simulink model "QuadcopterSimModel_INDI_Traj"  (R2018b)
settings: Solver=ode23  StartTime=0.0  StopTime=1000  FixedStep=sample_time  RelTol=1e-4  EnableMultiTasking=on
undefined symbols (not defined in the file): alt_ground, atmosphere, cycle, DiscIntNeverNeededParam, envir, fm_loiter, g, jystck, pos_ref, sigbuilder_block, traj_empty, waypoints, wind
libraries: simulink x6, ndi_lib x5, filters_lib x5, axes_transformation_lib x4, angles_lib x3, unit_conversions_lib x3, cntrl_atti_red_indi_lib x2, traj_lib x2, aerolibfltsims x2, control_allocation_lib x1, sensors_lib x1, atmosphere_lib x1
(part 1 of 3)
settings Model: Creator=Yannic  LastModifiedBy=eike
settings SolverCC: ZeroCrossControl=DisableAll
settings DataIOCC: LimitDataPoints=on  ReturnWorkspaceOutputs=on
settings OptimizationCC: EfficientMapNaN2IntZero=off  LifeSpan=inf
settings DebuggingCC: ReadBeforeWriteMsg=DisableAll  WriteAfterWriteMsg=DisableAll  WriteAfterReadMsg=DisableAll  MultiTaskDSMMsg=none  AllowSymbolicDim=off  LibraryContextMissingDiagnostic=none  SFUnexpectedBacktrackingDiag=warning  SFNoUnconditionalDefaultTransitionDiag=warning  SFExecutionAtInitializationDiag=none
settings HardwareCC: TargetBitPerLong=64  TargetBitPerPointer=64  TargetBitPerSizeT=64  TargetBitPerPtrDiffT=64  TargetLongLongMode=on  TargetIntDivRoundTo=Zero  TargetEndianess=LittleEndian  TargetWordSize=64  TargetHWDeviceType=MATLAB Host  ProdEqTarget=off
settings ModelReferenceCC: UpdateModelReferenceTargets=IfOutOfDate  PropagateSignalLabelsOutOfModel=off
settings SFSimCC: SFSimEcho=off  SimUseLocalCustomCode=off
settings CodeAppCC: MaxIdLength=128
settings GRTTargetCC: TargetLangStandard=C89/C90 (ANSI)  CombineOutputUpdateFcns=off  GRTInterface=on
settings ConfigComp: CovMetricSettings=dw  CovHtmlReporting=on  CovSaveCumulativeToWorkspaceVar=on  CovSaveSingleToWorkspaceVar=on  CovExternalEMLEnable=off

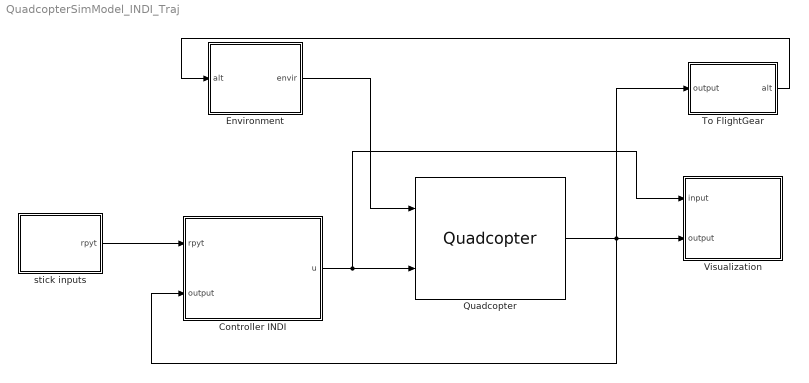
== system QuadcopterSimModel_INDI_Traj ==
  Controller INDI : Subsystem
  Environment : Subsystem
  Quadcopter : quadcopter_lib/Quadcopter  copter_=copter  IC_=IC  grnd_=grnd
      settings: SourceProductName=LADAC
  To FlightGear : Subsystem
  Visualization : Subsystem
  stick inputs : Subsystem
  wires:
  Environment/1(envir) -> Quadcopter/1
  Quadcopter/1 -> To FlightGear/1(output), Visualization/2(output), Controller INDI/2(output)
  To FlightGear/1(alt) -> Environment/1(alt)
  Controller INDI/1(u) -> Quadcopter/2, Visualization/1(input)
  stick inputs/1(rpyt) -> Controller INDI/1(rpyt)

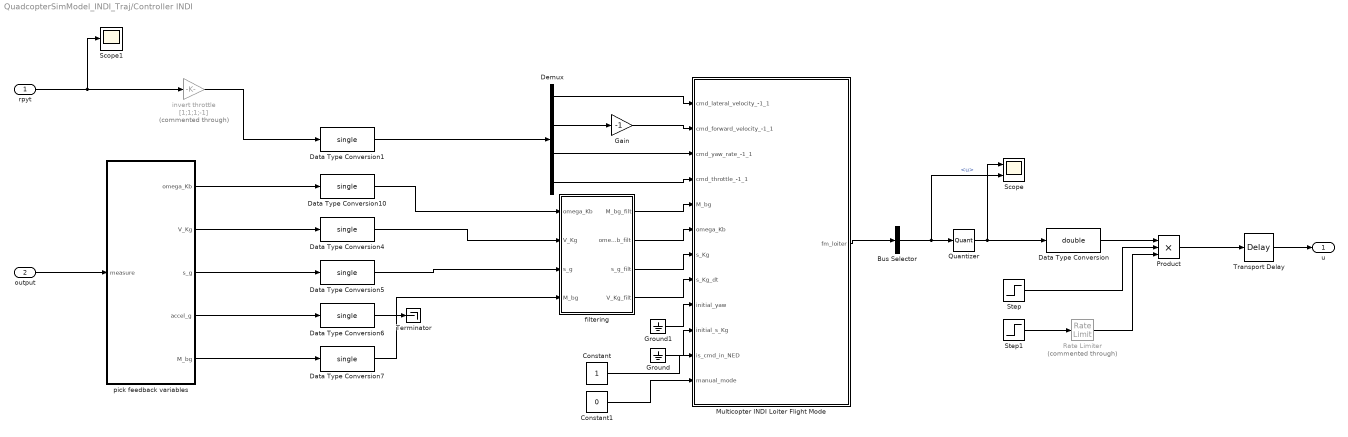
== system QuadcopterSimModel_INDI_Traj/Controller INDI ==
  rpyt : Inport  OutDataTypeStr=double
  output : Inport  Port=2
  Bus Selector : BusSelector  OutputSignals=fm_alt_hold.u
  Constant : Constant
  Constant1 : Constant  Value=0  OutDataTypeStr=single
  Data Type Conversion : DataTypeConversion  OutDataTypeStr=double
  Data Type Conversion{1,4..7,10} (6 alike) : DataTypeConversion  OutDataTypeStr=single
  Demux : Demux
  Gain : Gain  Gain=-1
  Ground : Ground
  Ground1 : Ground
  Multicopter INDI Loiter Flight Mode : Subsystem  AncestorBlock=fm_copter_loiter_indi_lib/Multicopter INDI Loiter Flight Mode  mask{fm=fm_loiter}
      mask prompts: fm "Multicopter INDI loiter flight  struct"
      mask DialogControl DescGroupVar Prompt: Multicopter INDI Loiter Flight Mode
      mask DialogControl DescTextVar Prompt: Loiter flight mode using the reduced attitude controller with INDI.
      mask DialogControl Control2 Prompt: To intialize the parameters struct see multicopterFlightModeLoiter.
  Product : Product  Inputs=3
  Quantizer : Quantizer  QuantizationInterval=0.001
  Rate Limiter : RateLimiter  Commented=through  SampleTimeMode=inherited  InitialCondition=1
  Scope : Scope  NumInputPorts=2
  Scope1 : Scope
  Step : Step  Time=100  Before=[1;1;1;1]  After=[1;1;1;1]  SampleTime=0
  Step1 : Step  Time=5  Before=[1;1;1;1]  After=[1;1;1;1]  SampleTime=0
  Terminator : Terminator
  Transport Delay : TransportDelay  DelayTime=0.01*0
  filtering : Subsystem
  invert throttle : Gain  Commented=through  Gain=[1;1;1;-1]
  pick feedback variables : Subsystem
  u : Outport  OutDataTypeStr=double  PortDimensions=4
  wires:
  pick feedback variables/1(omega_Kb) -> Data Type Conversion10/1
  output/1 -> pick feedback variables/1(measure)
  rpyt/1 -> invert throttle/1, Scope1/1
  Bus Selector/1 -> Scope/2, Quantizer/1  "<u>"
  pick feedback variables/3(s_g) -> Data Type Conversion5/1
  Data Type Conversion6/1 -> Terminator/1
  pick feedback variables/4(accel_g) -> Data Type Conversion6/1
  pick feedback variables/2(V_Kg) -> Data Type Conversion4/1
  Transport Delay/1 -> u/1
  Step/1 -> Product/2
  Data Type Conversion/1 -> Product/1
  Product/1 -> Transport Delay/1
  Rate Limiter/1 -> Product/3
  Data Type Conversion1/1 -> Demux/1
  pick feedback variables/5(M_bg) -> Data Type Conversion7/1
  Ground/1 -> Multicopter INDI Loiter Flight Mode/10(initial_s_Kg)
  Step1/1 -> Rate Limiter/1
  invert throttle/1 -> Data Type Conversion1/1
  Multicopter INDI Loiter Flight Mode/1(fm_loiter) -> Bus Selector/1
  Demux/4 -> Multicopter INDI Loiter Flight Mode/4(cmd_throttle_-1_1)
  Demux/3 -> Multicopter INDI Loiter Flight Mode/3(cmd_yaw_rate_-1_1)
  Constant/1 -> Multicopter INDI Loiter Flight Mode/11(is_cmd_in_NED)
  Ground1/1 -> Multicopter INDI Loiter Flight Mode/9(initial_yaw)
  Demux/2 -> Gain/1
  Demux/1 -> Multicopter INDI Loiter Flight Mode/1(cmd_lateral_velocity_-1_1)
  Gain/1 -> Multicopter INDI Loiter Flight Mode/2(cmd_forward_velocity_-1_1)
  Data Type Conversion10/1 -> filtering/1(omega_Kb)
  Data Type Conversion4/1 -> filtering/2(V_Kg)
  Data Type Conversion5/1 -> filtering/3(s_g)
  Data Type Conversion7/1 -> filtering/4(M_bg)
  filtering/1(M_bg_filt) -> Multicopter INDI Loiter Flight Mode/5(M_bg)
  filtering/2(omega_Kb_filt) -> Multicopter INDI Loiter Flight Mode/6(omega_Kb)
  filtering/3(s_g_filt) -> Multicopter INDI Loiter Flight Mode/7(s_Kg)
  filtering/4(V_Kg_filt) -> Multicopter INDI Loiter Flight Mode/8(s_Kg_dt)
  Quantizer/1 -> Scope/1, Data Type Conversion/1
  Constant1/1 -> Multicopter INDI Loiter Flight Mode/12(manual_mode)

== system QuadcopterSimModel_INDI_Traj/Environment ==
  alt : Inport
  Bus Assignment : BusAssignment  AssignedSignals=atmosphere,wind,g,alt_ground
  Bus Creator : BusCreator  Inputs=2
  Constant1 : Constant  Value=envir  OutDataTypeStr=Bus: envirBus
  Constant2 : Constant  Value=zeros(3,1)
  Constant3 : Constant  Value=envir.g
  From FlightGear : Subsystem
  Gain : Gain  Gain=0
  ISA Atmosphere Model : atmosphere_lib/ISA Atmosphere Model  SystemSampleTime=-1
      settings: SourceProductName=LADAC
  Rate Transition{,1..4} (5 alike) : RateTransition
  Step : Step  Time=5  After=[0;10;0]  SampleTime=0
  envir : Outport
  wires:
  From FlightGear/1(h_ground) -> Rate Transition1/1  "h"
  Rate Transition2/1 -> Bus Assignment/3
  Rate Transition3/1 -> Bus Assignment/2
  Bus Assignment/1 -> envir/1
  Rate Transition/1 -> Bus Assignment/1
  ISA Atmosphere Model/1 -> Rate Transition3/1
  Step/1 -> Gain/1  "V_Wg"
  Rate Transition1/1 -> Bus Assignment/5
  Constant1/1 -> Rate Transition/1
  alt/1 -> ISA Atmosphere Model/1
  Bus Creator/1 -> Rate Transition2/1
  Constant2/1 -> Bus Creator/2  "V_Wg_dt"
  Rate Transition4/1 -> Bus Assignment/4
  Constant3/1 -> Rate Transition4/1
  Gain/1 -> Bus Creator/1

== system QuadcopterSimModel_INDI_Traj/To FlightGear ==
  output : Inport
  Bus Selector1 : BusSelector  OutputSignals=rigidBodyBus.s_g_in_m,rigidBodyBus.EulerAngles_in_rad,motorBus.angular_velocity_in_rad_per_s
  Compare To Constant : simulink/Logic and Bit Operations/Compare To Constant  relop=<=  const=2*pi*1000  OutDataTypeStr=boolean
  Constant : Constant  Value=4
  Flight Gear Animation (Quadcopter) : flightgear_visualization_lib/Flight Gear Animation (Quadcopter)  inital_lat=pos_ref.lat  inital_long=pos_ref.lon  inital_height=pos_ref.alt  remoteURL=fg.remoteURL  remotePort=fg.remotePort
      settings: SourceProductName=LADAC
  Ground : Ground
  Integrator : Integrator  ExternalReset=rising
  Selector : Selector  InputPortWidth=3  IndexOptions=Index vector (dialog)  Indices=3  OutputSizes=1
  Unit Delay : UnitDelay  SampleTime=-1
  geographic position : Subsystem
  rad2deg : unit_conversions_lib/rad2deg
      settings: SourceProductName=LADAC
  alt : Outport
  wires:
  Bus Selector1/1 -> geographic position/1(s_E), Flight Gear Animation (Quadcopter)/1  "<s_g_in_m>"
  output/1 -> Bus Selector1/1
  geographic position/1(lat,lon,alt) -> Selector/1
  Bus Selector1/2 -> Flight Gear Animation (Quadcopter)/2  "<EulerAngles_in_rad>"
  Bus Selector1/3 -> rad2deg/1  "<angular_velocity_in_rad_per_s>"
  Selector/1 -> alt/1
  Constant/1 -> Flight Gear Animation (Quadcopter)/3
  Ground/1 -> Flight Gear Animation (Quadcopter)/4
  Integrator/1 -> Unit Delay/1, Flight Gear Animation (Quadcopter)/5
  Unit Delay/1 -> Compare To Constant/1
  Compare To Constant/1 -> Integrator/2
  rad2deg/1 -> Integrator/1

== system QuadcopterSimModel_INDI_Traj/Visualization ==
  input : Inport
  output : Inport  Port=2
  Aerodynamics : Subsystem
  Bus Selector : BusSelector  OutputSignals=rigidBodyBus,aeroBus,propulsionBus,motorBus
  Motor : Subsystem
  Propulsion : Subsystem
  Scope : Scope
  rigid_body : Subsystem
  wires:
  output/1 -> Bus Selector/1
  Bus Selector/1 -> rigid_body/1(rigidBodyBus)  "<rigidBodyBus>"
  Bus Selector/2 -> Aerodynamics/1(aeroBus)  "<aeroBus>"
  Bus Selector/3 -> Propulsion/1(propulsionBus)  "<propulsionBus>"
  Bus Selector/4 -> Motor/1(motorBus)  "<motorBus>"
  input/1 -> Scope/1

== system QuadcopterSimModel_INDI_Traj/stick inputs ==
  Calibrated Joystick : joystick_lib/Calibrated Joystick  jystck=jystck
      settings: SourceProductName=LADAC
  Constant1 : Constant  Value=jystck.enable
  Scope : Scope
  Selector2 : Selector  InputPortWidth=8  IndexOptions=Index vector (dialog)  Indices=[1,2,3,4]  OutputSizes=1
  Signal builder : Subsystem
  Switch1 : Switch  Criteria=u2 > Threshold
  rpyt : Outport
  wires:
  Signal builder/1(r) -> Switch1/3
  Switch1/1 -> Selector2/1, Scope/1
  Constant1/1 -> Calibrated Joystick/Enable, Switch1/2
  Calibrated Joystick/1 -> Switch1/1
  Selector2/1 -> rpyt/1

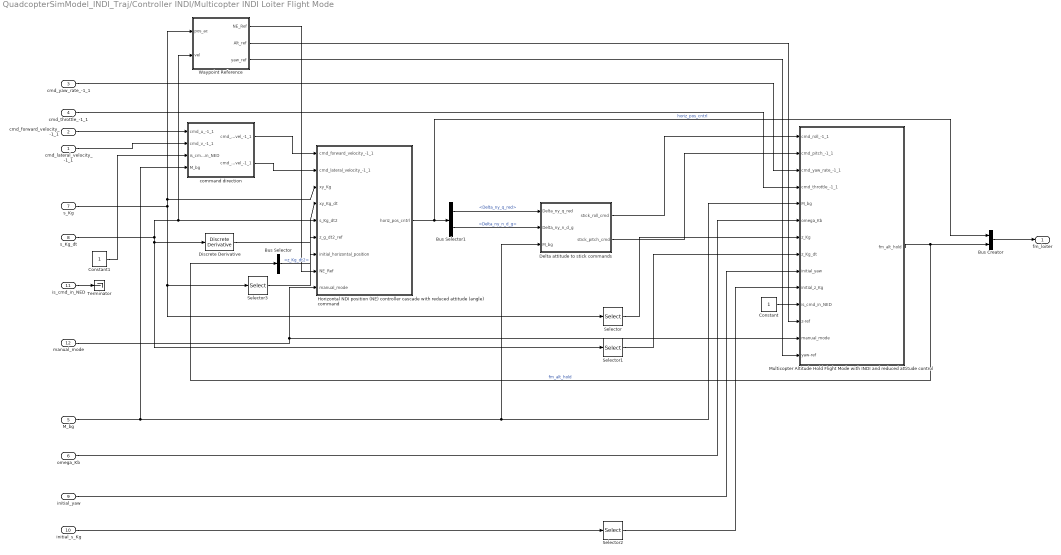
== system QuadcopterSimModel_INDI_Traj/Controller INDI/Multicopter INDI Loiter Flight Mode ==
  cmd_lateral_velocity_-1_1 : Inport  SampleTime=fm.sample_time
  cmd_forward_velocity_-1_1 : Inport  Port=2  SampleTime=fm.sample_time
  cmd_yaw_rate_-1_1 : Inport  Port=3  SampleTime=fm.sample_time
  cmd_throttle_-1_1 : Inport  Port=4  SampleTime=fm.sample_time
  M_bg : Inport  Port=5  SampleTime=fm.sample_time
  omega_Kb : Inport  Port=6  SampleTime=fm.sample_time
  s_Kg : Inport  Port=7  SampleTime=fm.sample_time
  s_Kg_dt : Inport  Port=8  SampleTime=fm.sample_time
  initial_yaw : Inport  Port=9  SampleTime=fm.sample_time
  initial_s_Kg : Inport  Port=10  SampleTime=fm.sample_time
  is_cmd_in_NED : Inport  Port=11  SampleTime=fm.sample_time
  manual_mode : Inport  Port=12
  Bus Creator : BusCreator  Inputs=2
  Bus Selector : BusSelector  OutputSignals=alt_cntrl.reference.z_Kg_dt2
  Bus Selector1 : BusSelector  OutputSignals=pseudo_control.Delta_ny_q_red,pseudo_control.Delta_ny_n_d_g
  Constant : Constant
  Constant1 : Constant  OutDataTypeStr=Inherit: Inherit via back propagation
  Delta attitude to stick commands : Subsystem
  Discrete Derivative : simulink/Discrete/Discrete Derivative  gainval=1.0  ICPrevScaledInput=0.0  OutMin=[]  OutMax=[]  OutDataType=fixdt(1, 16)  OutScaling=2^-10  DoSatur=off
  Horizontal NDI position (NE) controller cascade with reduced attitude (angle) command : Subsystem  AncestorBlock=|  mask{horiz_pos_cntrl=fm.horiz_pos_cntrl, T=2./fm.fm_alt.cntrl.atti_cntrl.rm.lean.omega + fm.fm_alt.motor_time_constant + 2./fm.fm_alt.sens_filt.omega}
      | cntrl_horiz_pos_indi_lib/Horizontal NDI position (NE) controller cascade
      | with reduced attitude (angle) command
      mask prompts: horiz_pos_cntrl "horizontal position controller struct"; T "inner loop time constant"
      mask DialogControl DescGroupVar Prompt: Horizontal position controller cascade
      mask DialogControl DescTextVar Prompt: The commanded velocity is filtered and the control error is converted into desired accerlations in x_g and y_g direction. The commanded accelerations are converted into commanded to reduced attitude angles.
      mask DialogControl Control2 Prompt: To initialize a horizontal position controller parameters struct see cntrlHorizPosIndiLoadParams
  Multicopter Altitude Hold Flight Mode with INDI and reduced attitude control : Subsystem  AncestorBlock=fm_copter_alt_hold_indi_lib/Multicopter Altitude Hold Flight Mode with INDI and reduced attitude control  mask{fm=fm.fm_alt}
      mask prompts: fm "Multicopter Altitude Hold Flight Mode (INDI) struct"
      mask DialogControl DescGroupVar Prompt: Multicopter Attitude Flight Mode with INDI and reduced attitude control
      mask DialogControl DescTextVar Prompt: Controller is basically implemented according to [1]
      mask DialogControl Control2 Prompt: [1] Sun, S., Baert, M., Van Schijndel, B. S., & De Visser, C. (2020, May). Upset Recovery Control for Quadrotors Subjected to a Complete Rotor Failure from Large Initial Disturbances. In 2020 IEEE International Conference on Robotics and Automation (ICRA) (pp. 4273-4279). IEEE.
      mask DialogControl Control3 Prompt: To initialize an altitude hold flight mode struct see fmCopterAltHoldIndiLoadParams
  Selector : Selector  InputPortWidth=3  IndexOptions=Index vector (dialog)  Indices=3  OutputSizes=1
  Selector1 : Selector  InputPortWidth=3  IndexOptions=Index vector (dialog)  Indices=3  OutputSizes=1
  Selector2 : Selector  InputPortWidth=3  IndexOptions=Index vector (dialog)  Indices=3  OutputSizes=1
  Selector3 : Selector  InputPortWidth=3  IndexOptions=Index vector (dialog)  Indices=[1,2]  OutputSizes=1
  Terminator : Terminator
  Waypoint Reference : Subsystem
  command direction : Subsystem
  fm_loiter : Outport  OutDataTypeStr=single  SampleTime=fm.sample_time
  wires:
  is_cmd_in_NED/1 -> Terminator/1
  command direction/2(cmd_east_vel_-1_1) -> Horizontal NDI position (NE) controller cascade with reduced attitude (angle) command/2(cmd_lateral_velocity_-1_1)
  command direction/1(cmd_north_vel_-1_1) -> Horizontal NDI position (NE) controller cascade with reduced attitude (angle) command/1(cmd_forward_velocity_-1_1)
  Bus Creator/1 -> fm_loiter/1
  Bus Selector1/1 -> Delta attitude to stick commands/1(Delta_ny_q_red)  "<Delta_ny_q_red>"
  Selector2/1 -> Multicopter Altitude Hold Flight Mode with INDI and reduced attitude control/10(initial_z_Kg)
  Constant1/1 -> command direction/3(is_cmd_in_NED)
  Delta attitude to stick commands/1(stick_roll_cmd) -> Multicopter Altitude Hold Flight Mode with INDI and reduced attitude control/1(cmd_roll_-1_1)
  Selector/1 -> Multicopter Altitude Hold Flight Mode with INDI and reduced attitude control/7(z_Kg)
  cmd_lateral_velocity_-1_1/1 -> command direction/2(cmd_v_-1_1)
  Bus Selector/1 -> Horizontal NDI position (NE) controller cascade with reduced attitude (angle) command/6(z_g_dt2_ref)  "<z_Kg_dt2>"
  cmd_throttle_-1_1/1 -> Multicopter Altitude Hold Flight Mode with INDI and reduced attitude control/4(cmd_throttle_-1_1)
  initial_yaw/1 -> Multicopter Altitude Hold Flight Mode with INDI and reduced attitude control/9(initial_yaw)
  Delta attitude to stick commands/2(stick_pitch_cmd) -> Multicopter Altitude Hold Flight Mode with INDI and reduced attitude control/2(cmd_pitch_-1_1)
  s_Kg/1 -> Selector/1, Selector3/1, Waypoint Reference/1(pos_ac), Horizontal NDI position (NE) controller cascade with reduced attitude (angle) command/3(xy_Kg)
  Selector1/1 -> Multicopter Altitude Hold Flight Mode with INDI and reduced attitude control/8(z_Kg_dt)
  Multicopter Altitude Hold Flight Mode with INDI and reduced attitude control/1(fm_alt_hold) -> Bus Selector/1, Bus Creator/2  "fm_alt_hold"
  M_bg/1 -> command direction/4(M_bg), Multicopter Altitude Hold Flight Mode with INDI and reduced attitude control/5(M_bg), Delta attitude to stick commands/3(M_bg)
  Bus Selector1/2 -> Delta attitude to stick commands/2(Delta_ny_n_d_g)  "<Delta_ny_n_d_g>"
  Horizontal NDI position (NE) controller cascade with reduced attitude (angle) command/1(horiz_pos_cntrl) -> Bus Selector1/1, Bus Creator/1  "horiz_pos_cntrl"
  omega_Kb/1 -> Multicopter Altitude Hold Flight Mode with INDI and reduced attitude control/6(omega_Kb)
  initial_s_Kg/1 -> Selector2/1
  Selector3/1 -> Horizontal NDI position (NE) controller cascade with reduced attitude (angle) command/7(initial_horizontal_position)
  Constant/1 -> Multicopter Altitude Hold Flight Mode with INDI and reduced attitude control/11(is_cmd_in_NED)
  cmd_yaw_rate_-1_1/1 -> Multicopter Altitude Hold Flight Mode with INDI and reduced attitude control/3(cmd_yaw_rate_-1_1)
  Discrete Derivative/1 -> Horizontal NDI position (NE) controller cascade with reduced attitude (angle) command/5(s_Kg_dt2)
  s_Kg_dt/1 -> Selector1/1, Discrete Derivative/1, Horizontal NDI position (NE) controller cascade with reduced attitude (angle) command/4(xy_Kg_dt), Waypoint Reference/2(vel)
  cmd_forward_velocity_-1_1/1 -> command direction/1(cmd_u_-1_1)
  Waypoint Reference/1(NE_Ref) -> Horizontal NDI position (NE) controller cascade with reduced attitude (angle) command/8(NE_Ref)
  manual_mode/1 -> Horizontal NDI position (NE) controller cascade with reduced attitude (angle) command/9(manual_mode), Multicopter Altitude Hold Flight Mode with INDI and reduced attitude control/13(manual_mode)
  Waypoint Reference/2(Alt_ref) -> Multicopter Altitude Hold Flight Mode with INDI and reduced attitude control/12(z-ref)
  Waypoint Reference/3(yaw_ref) -> Multicopter Altitude Hold Flight Mode with INDI and reduced attitude control/14(yaw-ref)

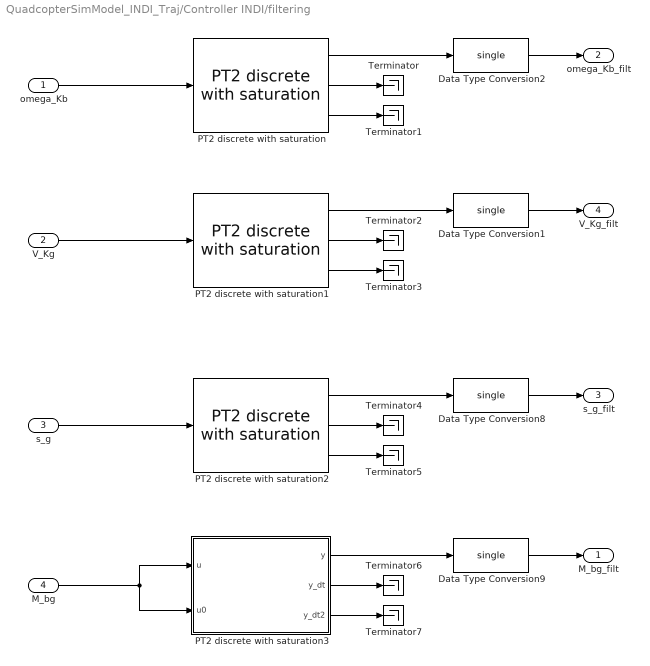
== system QuadcopterSimModel_INDI_Traj/Controller INDI/filtering ==
  omega_Kb : Inport
  V_Kg : Inport  Port=2
  s_g : Inport  Port=3
  M_bg : Inport  Port=4
  Data Type Conversion{1..2,8..9} (4 alike) : DataTypeConversion  OutDataTypeStr=single
  PT2 discrete with saturation : filters_lib/PT2 discrete with saturation  omega=fm_loiter.fm_alt.sens_filt.omega  d=fm_loiter.fm_alt.sens_filt.D  x_dt2_max=inf  x_dt2_min=-inf  x_dt_max=inf  x_dt_min=-inf  x_max=inf  x_min=-inf  x_init=0  x_dt_init=0
      settings: SourceProductName=LADAC
  PT2 discrete with saturation1 : filters_lib/PT2 discrete with saturation  omega=fm_loiter.sens_filt.omega  d=fm_loiter.sens_filt.D  x_dt2_max=inf  x_dt2_min=-inf  x_dt_max=inf  x_dt_min=-inf  x_max=inf  x_min=-inf  x_init=0  x_dt_init=0
      settings: SourceProductName=LADAC
  PT2 discrete with saturation2 : filters_lib/PT2 discrete with saturation  omega=fm_loiter.sens_filt.omega  d=fm_loiter.sens_filt.D  x_dt2_max=inf  x_dt2_min=-inf  x_dt_max=inf  x_dt_min=-inf  x_max=inf  x_min=-inf  x_init=0  x_dt_init=0
      settings: SourceProductName=LADAC
  PT2 discrete with saturation3 : Subsystem  mask{omega=fm_loiter.fm_alt.sens_filt.omega, d=fm_loiter.fm_alt.sens_filt.D, x_dt2_max=inf, x_dt2_min=-inf, x_dt_max=inf, x_dt_min=-inf, x_max=inf, x_min=-inf, x_init=0, x_dt_init=0}
      mask prompts: omega "Natural frequency"; d "Damping ratio"; x_dt2_max "Maximum acceleration"; x_dt2_min "Minimum acceleration"; x_dt_max "Maximum rate"; x_dt_min "Minimum rate"; x_max "Maximum position"; x_min "Minimum position"; x_init "Initial position"; x_dt_init "Initial rate"
  Terminator{,1..7} (8 alike) : Terminator
  M_bg_filt : Outport
  omega_Kb_filt : Outport  Port=2
  s_g_filt : Outport  Port=3
  V_Kg_filt : Outport  Port=4
  wires:
  omega_Kb/1 -> PT2 discrete with saturation/1
  PT2 discrete with saturation/1 -> Data Type Conversion2/1
  V_Kg/1 -> PT2 discrete with saturation1/1
  PT2 discrete with saturation1/1 -> Data Type Conversion1/1
  s_g/1 -> PT2 discrete with saturation2/1
  PT2 discrete with saturation2/1 -> Data Type Conversion8/1
  M_bg/1 -> PT2 discrete with saturation3/2(u0), PT2 discrete with saturation3/1(u)
  PT2 discrete with saturation3/1(y) -> Data Type Conversion9/1
  PT2 discrete with saturation/2 -> Terminator/1
  PT2 discrete with saturation/3 -> Terminator1/1
  PT2 discrete with saturation1/2 -> Terminator2/1
  PT2 discrete with saturation1/3 -> Terminator3/1
  PT2 discrete with saturation2/2 -> Terminator4/1
  PT2 discrete with saturation2/3 -> Terminator5/1
  PT2 discrete with saturation3/2(y_dt) -> Terminator6/1
  PT2 discrete with saturation3/3(y_dt2) -> Terminator7/1
  Data Type Conversion9/1 -> M_bg_filt/1
  Data Type Conversion8/1 -> s_g_filt/1
  Data Type Conversion1/1 -> V_Kg_filt/1
  Data Type Conversion2/1 -> omega_Kb_filt/1

== system QuadcopterSimModel_INDI_Traj/Controller INDI/pick feedback variables ==
  measure : Inport
  Bus Selector1 : BusSelector  OutputSignals=rigidBodyBus.omega_Kb_in_rad_per_s,rigidBodyBus.EulerAngles_in_rad,rigidBodyBus.V_Kg_in_m_per_s,rigidBodyBus.s_g_in_m,rigidBodyBus.dot_V_Kb_in_m_per_square_s,rigidBodyBus.V_Kb_m_per_s,rigidBodyBus.M_bg_in_1
  Constant : Constant  Value=envir.g  OutDataTypeStr=Inherit: Inherit via back propagation
  Euler Angles to Rotation Matrix : axes_transformation_lib/Euler Angles to Rotation Matrix  SystemSampleTime=-1
      settings: SourceProductName=LADAC
  Matrix Multiply : Product  Multiplication=Matrix(*)
  Transpose : Math  Operator=transpose  SaturateOnIntegerOverflow=on
  accelerometer : sensors_lib/accelerometer  SystemSampleTime=-1
  omega_Kb : Outport
  V_Kg : Outport  Port=2
  s_g : Outport  Port=3
  accel_g : Outport  Port=4
  M_bg : Outport  Port=5
  wires:
  measure/1 -> Bus Selector1/1
  Bus Selector1/3 -> V_Kg/1  "<V_Kg_in_m_per_s>"
  Bus Selector1/2 -> Euler Angles to Rotation Matrix/1  "<EulerAngles_in_rad>"
  Bus Selector1/1 -> omega_Kb/1, accelerometer/3  "<omega_Kb_in_rad_per_s>"
  Bus Selector1/4 -> s_g/1  "<s_g_in_m>"
  Bus Selector1/5 -> accelerometer/1  "<dot_V_Kb_in_m_per_square_s>"
  Euler Angles to Rotation Matrix/1 -> accelerometer/4, Transpose/1
  Bus Selector1/6 -> accelerometer/2  "<V_Kb_m_per_s>"
  Constant/1 -> accelerometer/5
  accelerometer/1 -> Matrix Multiply/2
  Matrix Multiply/1 -> accel_g/1
  Transpose/1 -> Matrix Multiply/1
  Bus Selector1/7 -> M_bg/1  "<M_bg_in_1>"

== system QuadcopterSimModel_INDI_Traj/Environment/From FlightGear ==
  Receive net_ctrl Packet from FlightGear : aerolibfltsims/Receive net_ctrl Packet from FlightGear  FlightGearVersion=v3.4  ReceiveAddress=127.0.0.1  ReceivePort=5503  ReceiveWidth=744  varLen=off  SampleTime=1/5  packetFlag=on
      settings: AttributesFormatString=Version Selected:\n%<FlightGearVersion>  SourceProductName=Aerospace Blockset  SourceProductBaseCode=AE
  Scope : Scope
  Scope1 : Scope
  Terminator{,1..6} (7 alike) : Terminator
  Unpack net_ctrl Packet from FlightGear : aerolibfltsims/Unpack net_ctrl Packet from FlightGear  FlightGearVersion=v3.4  ShowControlSurfacePositionOutputs=off  ShowEngineFuelOutputs=off  ShowLandingGearOutputs=off  ShowAvionicOutputs=off  ShowEnvironmentOutputs=on  SampleTime=1/5  packetVersion=27
      settings: AttributesFormatString=Version Selected: %<FlightGearVersion>  SourceProductName=Aerospace Blockset  SourceProductBaseCode=AE
  h_ground : Outport
  wires:
  Unpack net_ctrl Packet from FlightGear/4 -> Terminator3/1
  Unpack net_ctrl Packet from FlightGear/5 -> Terminator4/1
  Receive net_ctrl Packet from FlightGear/1 -> Unpack net_ctrl Packet from FlightGear/1
  Unpack net_ctrl Packet from FlightGear/2 -> Terminator1/1
  Unpack net_ctrl Packet from FlightGear/7 -> Terminator5/1
  Unpack net_ctrl Packet from FlightGear/1 -> Terminator/1
  Unpack net_ctrl Packet from FlightGear/3 -> Terminator2/1
  Unpack net_ctrl Packet from FlightGear/8 -> Terminator6/1
  Unpack net_ctrl Packet from FlightGear/6 -> Scope/1, h_ground/1
  Receive net_ctrl Packet from FlightGear/2 -> Scope1/1

== system QuadcopterSimModel_INDI_Traj/To FlightGear/geographic position ==
  s_E : Inport
  Constant : Constant  Value=pos_ref.lat
  Constant1 : Constant  Value=pos_ref.lon
  Constant2 : Constant  Value=pos_ref.alt
  Mux : Mux  Inputs=3
  Scope : Scope  NumInputPorts=3
  "flat earth to lat, lon, alt" : axes_transformation_lib/NED to lat, lon, alt  SystemSampleTime=-1
      settings: SourceProductName=LADAC
  lat,lon,alt : Outport
  wires:
  Constant2/1 -> "flat earth to lat, lon, alt"/3
  Constant1/1 -> "flat earth to lat, lon, alt"/2
  "flat earth to lat, lon, alt"/3 -> Scope/3, Mux/3
  Constant/1 -> "flat earth to lat, lon, alt"/1
  Mux/1 -> lat,lon,alt/1
  s_E/1 -> "flat earth to lat, lon, alt"/4
  "flat earth to lat, lon, alt"/2 -> Mux/2, Scope/2
  "flat earth to lat, lon, alt"/1 -> Mux/1, Scope/1

== system QuadcopterSimModel_INDI_Traj/Visualization/Aerodynamics ==
  aeroBus : Inport
  Bus Selector : BusSelector  OutputSignals=V_Ab_in_m_per_s,V_A_in_m_per_s,q_in_Pa,angles.alpha_M_in_rad,angles.beta_M_in_rad,M_ba_in_1,R_Ab_in_N,Q_Ab_in_N_m
  Scope{,1..6} (7 alike) : Scope
  Terminator : Terminator
  wires:
  aeroBus/1 -> Bus Selector/1
  Bus Selector/1 -> Scope/1  "<V_Ab_in_m_per_s>"
  Bus Selector/2 -> Scope1/1  "<V_A_in_m_per_s>"
  Bus Selector/3 -> Scope2/1  "<q_in_Pa>"
  Bus Selector/4 -> Scope3/1  "<alpha_M_in_rad>"
  Bus Selector/5 -> Scope4/1  "<beta_M_in_rad>"
  Bus Selector/6 -> Terminator/1  "<M_ba_in_1>"
  Bus Selector/7 -> Scope5/1  "<R_Ab_in_N>"
  Bus Selector/8 -> Scope6/1  "<Q_Ab_in_N_m>"

== system QuadcopterSimModel_INDI_Traj/Visualization/Motor ==
  motorBus : Inport
  Bus Selector : BusSelector  OutputSignals=angular_acceleration_in_rad_per_square_s,angular_velocity_in_rad_per_s
  Scope : Scope
  Scope1 : Scope
  wires:
  Bus Selector/1 -> Scope/1  "<angular_acceleration_in_rad_per_square_s>"
  motorBus/1 -> Bus Selector/1
  Bus Selector/2 -> Scope1/1  "<angular_velocity_in_rad_per_s>"

== system QuadcopterSimModel_INDI_Traj/Visualization/Propulsion ==
  propulsionBus : Inport
  Bus Selector : BusSelector  OutputSignals=propeller_1.thrust_in_N,propeller_2.thrust_in_N,propeller_3.thrust_in_N,propeller_4.thrust_in_N,propeller_1.torque_in_N,propeller_2.torque_in_N,propeller_3.torque_in_N,propeller_4.torque_in_N,propeller_1.R_Fb_in_N,propeller_2.R_Fb_in_N,propeller_3.R_Fb_in_N,propeller_4.R_Fb_in_N,propeller_1.Q_Fb_in_Nm,propeller_2.Q_Fb_in_Nm,propeller_3.Q_Fb_in_Nm,propeller_4.Q_Fb_in_Nm,propeller_1.V_A_prop_in_m_per_s,propeller_2.V_A_prop_in_m_per_s,propeller_3.V_A_prop_in_m_per_s,propeller_4.V_A_prop_in_m_per_s,R_Fb_in_N,Q_Fb_in_N
  Q_Fb : Scope  NumInputPorts=4
  R_Fb : Scope  NumInputPorts=4
  Scope5 : Scope
  Scope6 : Scope
  V_A_prop : Scope  NumInputPorts=4
  thrust : Scope  NumInputPorts=4
  torque : Scope  NumInputPorts=4
  wires:
  propulsionBus/1 -> Bus Selector/1
  Bus Selector/1 -> thrust/1  "<thrust_in_N>"
  Bus Selector/2 -> thrust/2  "<thrust_in_N>"
  Bus Selector/3 -> thrust/3  "<thrust_in_N>"
  Bus Selector/4 -> thrust/4  "<thrust_in_N>"
  Bus Selector/5 -> torque/1  "<torque_in_N>"
  Bus Selector/6 -> torque/2  "<torque_in_N>"
  Bus Selector/7 -> torque/3  "<torque_in_N>"
  Bus Selector/8 -> torque/4  "<torque_in_N>"
  Bus Selector/9 -> R_Fb/1  "<R_Fb_in_N>"
  Bus Selector/10 -> R_Fb/2  "<R_Fb_in_N>"
  Bus Selector/11 -> R_Fb/3  "<R_Fb_in_N>"
  Bus Selector/12 -> R_Fb/4  "<R_Fb_in_N>"
  Bus Selector/13 -> Q_Fb/1  "<Q_Fb_in_Nm>"
  Bus Selector/14 -> Q_Fb/2  "<Q_Fb_in_Nm>"
  Bus Selector/15 -> Q_Fb/3  "<Q_Fb_in_Nm>"
  Bus Selector/16 -> Q_Fb/4  "<Q_Fb_in_Nm>"
  Bus Selector/17 -> V_A_prop/1  "<V_A_prop_in_m_per_s>"
  Bus Selector/18 -> V_A_prop/2  "<V_A_prop_in_m_per_s>"
  Bus Selector/19 -> V_A_prop/3  "<V_A_prop_in_m_per_s>"
  Bus Selector/20 -> V_A_prop/4  "<V_A_prop_in_m_per_s>"
  Bus Selector/21 -> Scope5/1  "<R_Fb_in_N>"
  Bus Selector/22 -> Scope6/1  "<Q_Fb_in_N>"

== system QuadcopterSimModel_INDI_Traj/Visualization/rigid_body ==
  rigidBodyBus : Inport
  Bus Selector1 : BusSelector  OutputSignals=dot_V_Kb_in_m_per_square_s,dot_omega_Kb_in_rad_per_square_s,omega_Kb_in_rad_per_s,dot_q_bg_in_1_per_s,q_bg_in_1,EulerAngles_in_rad,dot_s_g_in_m,M_bg_in_1,V_Kg_in_m_per_s,V_Kb_m_per_s,s_g_in_m
  Demux : Demux  Outputs=3
  Demux1 : Demux  Outputs=3
  Demux2 : Demux  Outputs=3
  Phi,Theta,Psi : Scope  NumInputPorts=3
  Scope1 : Scope
  Scope2 : Scope
  Terminator{,1..5} (6 alike) : Terminator
  V_Kb : Scope  NumInputPorts=3
  p,q,r : Scope  NumInputPorts=3
  rad2deg : unit_conversions_lib/rad2deg
      settings: SourceProductName=LADAC
  rad2deg1 : unit_conversions_lib/rad2deg
      settings: SourceProductName=LADAC
  wires:
  Demux/1 -> p,q,r/1  "p (deg/s)"
  Demux1/2 -> Phi,Theta,Psi/2  "Theta (deg)"
  rad2deg/1 -> Demux/1
  Demux1/1 -> Phi,Theta,Psi/1  "Phi (deg)"
  Demux1/3 -> Phi,Theta,Psi/3  "Psi (deg)"
  Demux2/3 -> V_Kb/3  "w_Kb (m/s)"
  Bus Selector1/7 -> Terminator4/1  "<dot_s_g_in_m>"
  Bus Selector1/6 -> rad2deg1/1  "<EulerAngles_in_rad>"
  Bus Selector1/3 -> rad2deg/1  "<omega_Kb_in_rad_per_s>"
  Demux/3 -> p,q,r/3  "r (deg/s)"
  Bus Selector1/1 -> Terminator/1  "<dot_V_Kb_in_m_per_square_s>"
  Demux2/2 -> V_Kb/2  "v_Kb (m/s)"
  Demux/2 -> p,q,r/2  "q (deg/s)"
  rad2deg1/1 -> Demux1/1
  Bus Selector1/5 -> Terminator3/1  "<q_bg_in_1>"
  Demux2/1 -> V_Kb/1  "u_Kb (m/s)"
  Bus Selector1/10 -> Demux2/1  "<V_Kb_m_per_s>"
  rigidBodyBus/1 -> Bus Selector1/1
  Bus Selector1/8 -> Terminator5/1  "<M_bg_in_1>"
  Bus Selector1/4 -> Terminator2/1  "<dot_q_bg_in_1_per_s>"
  Bus Selector1/2 -> Terminator1/1  "<dot_omega_Kb_in_rad_per_square_s>"
  Bus Selector1/9 -> Scope2/1  "<V_Kg_in_m_per_s>"
  Bus Selector1/11 -> Scope1/1  "<s_g_in_m>"

== system QuadcopterSimModel_INDI_Traj/stick inputs/Signal builder ==
  Gain : Gain  Gain=0.5
  Gain1 : Gain  Gain=-0.5
  Gain2 : Gain  Gain=0.5
  Ground{,1..3} (4 alike) : Ground
  Mux2 : Mux  Inputs=8
  Selector2 : Selector  InputPortWidth=8  IndexOptions=Index vector (dialog)  Indices=[3,4,1,2,5,6,7,8]  OutputSizes=1
  Signal Builder : Subsystem  Tag=STV Subsys  LoadFcn=sigbuilder_block('load');  StartFcn=sigbuilder_block('start');  StopFcn=sigbuilder_block('stop');  ClipboardFcn=sigbuilder_block('clipboard');  mask(Sigbuilder block){tuvar=[0:10]}
      mask help: Simulink:masks:SigbuilderBlock_MD
      mask init:
      | if ~strcmp(get_param(bdroot(gcbh),'SimulationStatus'),'stopped') tuvar = sigbuilder_block('maskInit'); end
      settings: CopyFcn=sigbuilder_block('copy');  DeleteFcn=sigbuilder_block('delete');  ModelCloseFcn=sigbuilder_block('modelClose');  PreSaveFcn=sigbuilder_block('preSave');  PauseFcn=sigbuilder_block('pause');  ContinueFcn=sigbuilder_block('continue');  NameChangeFcn=sigbuilder_block('namechange');  OpenFcn=sigbuilder_block('open',[426 42.75 821.25 509.25 ]);  CloseFcn=sigbuilder_block('close');
      mask Display: plot(0, 0, 100, 100,[2, 2, 32, 32, 2], [68, 8, 8, 68, 68],[32, 2], [38, 38], [32, 19, 2],[53, 60, 44], [32, 17, 17, 2],[16, 16, 31, 31]);txt = getActiveGroup(gcbh);text(2, 100, txt,'verticalAlignment', 'top');
  Signal Builder1 : Subsystem  Tag=STV Subsys  LoadFcn=sigbuilder_block('load');  StartFcn=sigbuilder_block('start');  StopFcn=sigbuilder_block('stop');  ClipboardFcn=sigbuilder_block('clipboard');  mask(Sigbuilder block){tuvar=[0:10]}
      mask help: Simulink:masks:SigbuilderBlock_MD
      mask init:
      | if ~strcmp(get_param(bdroot(gcbh),'SimulationStatus'),'stopped') tuvar = sigbuilder_block('maskInit'); end
      settings: CopyFcn=sigbuilder_block('copy');  DeleteFcn=sigbuilder_block('delete');  ModelCloseFcn=sigbuilder_block('modelClose');  PreSaveFcn=sigbuilder_block('preSave');  PauseFcn=sigbuilder_block('pause');  ContinueFcn=sigbuilder_block('continue');  NameChangeFcn=sigbuilder_block('namechange');  OpenFcn=sigbuilder_block('open',[429.75 123 565.5 444.75 ]);  CloseFcn=sigbuilder_block('close');
      mask Display: plot(0, 0, 100, 100,[2, 2, 32, 32, 2], [68, 8, 8, 68, 68],[32, 2], [38, 38], [32, 19, 2],[53, 60, 44], [32, 17, 17, 2],[16, 16, 31, 31]);txt = getActiveGroup(gcbh);text(2, 100, txt,'verticalAlignment', 'top');
  Signal Builder2 : Subsystem  Tag=STV Subsys  LoadFcn=sigbuilder_block('load');  StartFcn=sigbuilder_block('start');  StopFcn=sigbuilder_block('stop');  ClipboardFcn=sigbuilder_block('clipboard');  mask(Sigbuilder block){tuvar=[0:10]}
      mask help: Simulink:masks:SigbuilderBlock_MD
      mask init:
      | if ~strcmp(get_param(bdroot(gcbh),'SimulationStatus'),'stopped') tuvar = sigbuilder_block('maskInit'); end
      settings: CopyFcn=sigbuilder_block('copy');  DeleteFcn=sigbuilder_block('delete');  ModelCloseFcn=sigbuilder_block('modelClose');  PreSaveFcn=sigbuilder_block('preSave');  PauseFcn=sigbuilder_block('pause');  ContinueFcn=sigbuilder_block('continue');  NameChangeFcn=sigbuilder_block('namechange');  OpenFcn=sigbuilder_block('open',[411 0 603 557.25 ]);  CloseFcn=sigbuilder_block('close');
      mask Display: plot(0, 0, 100, 100,[2, 2, 32, 32, 2], [68, 8, 8, 68, 68],[32, 2], [38, 38], [32, 19, 2],[53, 60, 44], [32, 17, 17, 2],[16, 16, 31, 31]);txt = getActiveGroup(gcbh);text(2, 100, txt,'verticalAlignment', 'top');
  Signal Builder3 : Subsystem  Tag=STV Subsys  LoadFcn=sigbuilder_block('load');  StartFcn=sigbuilder_block('start');  StopFcn=sigbuilder_block('stop');  ClipboardFcn=sigbuilder_block('clipboard');  mask(Sigbuilder block){tuvar=[0:10]}
      mask help: Simulink:masks:SigbuilderBlock_MD
      mask init:
      | if ~strcmp(get_param(bdroot(gcbh),'SimulationStatus'),'stopped') tuvar = sigbuilder_block('maskInit'); end
      settings: CopyFcn=sigbuilder_block('copy');  DeleteFcn=sigbuilder_block('delete');  ModelCloseFcn=sigbuilder_block('modelClose');  PreSaveFcn=sigbuilder_block('preSave');  PauseFcn=sigbuilder_block('pause');  ContinueFcn=sigbuilder_block('continue');  NameChangeFcn=sigbuilder_block('namechange');  OpenFcn=sigbuilder_block('open',[433.5 161.25 558 422.25 ]);  CloseFcn=sigbuilder_block('close');
      mask Display: plot(0, 0, 100, 100,[2, 2, 32, 32, 2], [68, 8, 8, 68, 68],[32, 2], [38, 38], [32, 19, 2],[53, 60, 44], [32, 17, 17, 2],[16, 16, 31, 31]);txt = getActiveGroup(gcbh);text(2, 100, txt,'verticalAlignment', 'top');
  r : Outport
  wires:
  Ground3/1 -> Mux2/8
  Gain2/1 -> Mux2/1  "LS_LR_-1,1"
  Ground1/1 -> Mux2/6
  Ground2/1 -> Mux2/7
  Mux2/1 -> Selector2/1
  Signal Builder2/1(Signal 1) -> Mux2/2  "LS_UD_-1,1"
  Gain/1 -> Mux2/3  "RS_LR_-1,1"
  Ground/1 -> Mux2/5
  Gain1/1 -> Mux2/4  "RS_DU_-1,1"
  Signal Builder3/1(Signal 1) -> Gain/1  "RS_LR_-1,1"
  Signal Builder/1(Signal 1) -> Gain1/1  "RS_DU_-1,1"
  Signal Builder1/1(Signal 1) -> Gain2/1  "LS_LR_-1,1"
  Selector2/1 -> r/1

== system QuadcopterSimModel_INDI_Traj/Controller INDI/Multicopter INDI Loiter Flight Mode/Delta attitude to stick commands ==
  Delta_ny_q_red : Inport
  Delta_ny_n_d_g : Inport  Port=2
  M_bg : Inport  Port=3
  Gain : Gain  Gain=1/fm.fm_alt.cntrl.atti_cntrl.rm.lean.max
  MATLAB Function1 : MATLAB Function  TreatAsAtomicUnit=on
  Saturation : Saturate  UpperLimit=fm.fm_alt.cntrl.atti_cntrl.rm.lean.max  LowerLimit=0
  conversion to total attitude command : Subsystem
  stick_roll_cmd : Outport
  stick_pitch_cmd : Outport  Port=2
  wires:
  Gain/1 -> MATLAB Function1/1(lean_angle_0_1)
  M_bg/1 -> conversion to total attitude command/3(M_bg)
  Delta_ny_q_red/1 -> conversion to total attitude command/1(Delta_q)
  Delta_ny_n_d_g/1 -> conversion to total attitude command/2(Delta_n_g)
  MATLAB Function1/2(stick_pitch_cmd) -> stick_pitch_cmd/1
  MATLAB Function1/1(stick_roll_cmd) -> stick_roll_cmd/1
  conversion to total attitude command/1(lean_angle) -> Saturation/1
  conversion to total attitude command/2(lean_direction_angle) -> MATLAB Function1/2(lean_direction_angle)
  Saturation/1 -> Gain/1

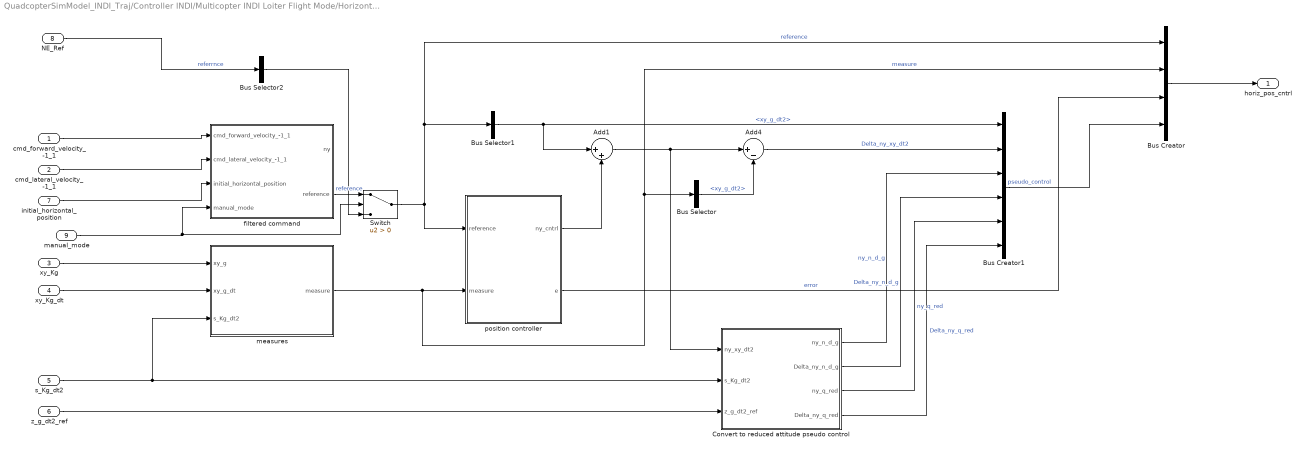
== system QuadcopterSimModel_INDI_Traj/Controller INDI/Multicopter INDI Loiter Flight Mode/Horizontal NDI position (NE) controller cascade with reduced attitude (angle) command ==
  cmd_forward_velocity_-1_1 : Inport
  cmd_lateral_velocity_-1_1 : Inport  Port=2
  xy_Kg : Inport  Port=3
  xy_Kg_dt : Inport  Port=4
  s_Kg_dt2 : Inport  Port=5
  z_g_dt2_ref : Inport  Port=6
  initial_horizontal_position : Inport  Port=7
  NE_Ref : Inport  Port=8
  manual_mode : Inport  Port=9
  Add1 : Sum  Inputs=|++
  Add4 : Sum  Inputs=|+-
  Bus Creator : BusCreator  Inputs=4
  Bus Creator1 : BusCreator  Inputs=6
  Bus Selector : BusSelector  OutputSignals=xy_g_dt2
  Bus Selector1 : BusSelector  OutputSignals=xy_g_dt2
  Bus Selector2 : BusSelector  OutputSignals=xy_g,xy_g_dt,xy_g_dt2  OutputAsBus=on
  Convert to reduced attitude pseudo control : Subsystem
  Switch : Switch  Criteria=u2 > Threshold
  filtered command : Subsystem
  measures : Subsystem
  position controller : Subsystem
  horiz_pos_cntrl : Outport
  wires:
  Convert to reduced attitude pseudo control/4(Delta_ny_q_red) -> Bus Creator1/6  "Delta_ny_q_red"
  Convert to reduced attitude pseudo control/3(ny_q_red) -> Bus Creator1/5  "ny_q_red"
  Convert to reduced attitude pseudo control/2(Delta_ny_n_d_g) -> Bus Creator1/4  "Delta_ny_n_d_g"
  Convert to reduced attitude pseudo control/1(ny_n_d_g) -> Bus Creator1/3  "ny_n_d_g"
  z_g_dt2_ref/1 -> Convert to reduced attitude pseudo control/3(z_g_dt2_ref)
  Bus Creator/1 -> horiz_pos_cntrl/1
  Bus Creator1/1 -> Bus Creator/4  "pseudo_control"
  Bus Selector/1 -> Add4/2  "<xy_g_dt2>"
  Add4/1 -> Bus Creator1/2  "Delta_ny_xy_dt2"
  measures/1(measure) -> position controller/2(measure), Bus Selector/1, Bus Creator/2  "measure"
  cmd_lateral_velocity_-1_1/1 -> filtered command/2(cmd_lateral_velocity_-1_1)
  xy_Kg_dt/1 -> measures/2(xy_g_dt)
  xy_Kg/1 -> measures/1(xy_g)
  position controller/2(e) -> Bus Creator/3  "error"
  s_Kg_dt2/1 -> Convert to reduced attitude pseudo control/2(s_Kg_dt2), measures/3(s_Kg_dt2)
  Add1/1 -> Add4/1, Convert to reduced attitude pseudo control/1(ny_xy_dt2)
  position controller/1(ny_cntrl) -> Add1/2
  initial_horizontal_position/1 -> filtered command/3(initial_horizontal_position)
  Switch/1 -> Bus Creator/1, Bus Selector1/1, position controller/1(reference)  "reference"
  cmd_forward_velocity_-1_1/1 -> filtered command/1(cmd_forward_velocity_-1_1)
  Bus Selector1/1 -> Add1/1, Bus Creator1/1  "<xy_g_dt2>"
  NE_Ref/1 -> Bus Selector2/1  "referrnce"
  Bus Selector2/1 -> Switch/3
  filtered command/2(reference) -> Switch/1  "reference"
  manual_mode/1 -> filtered command/4(manual_mode), Switch/2

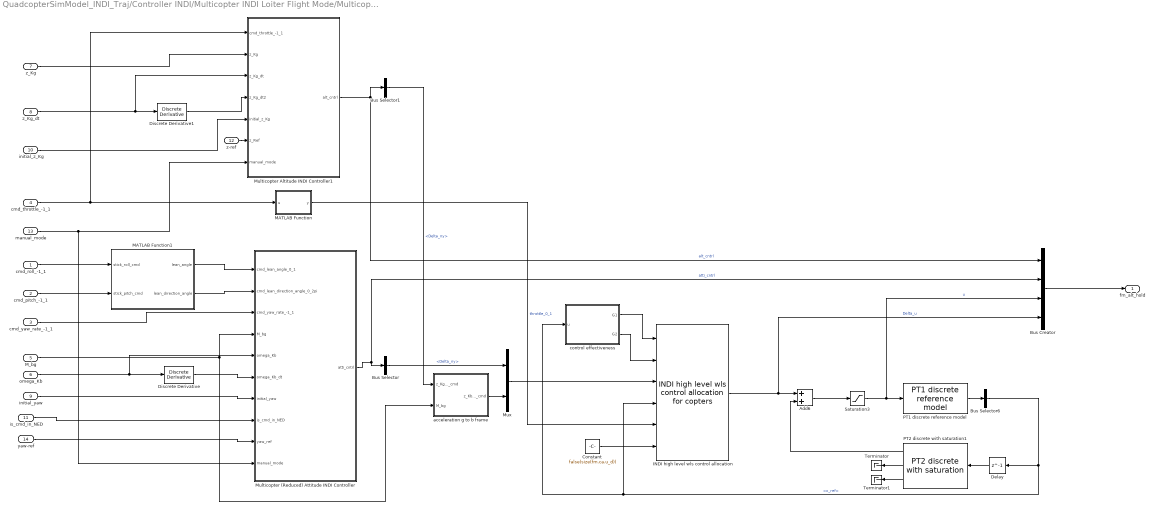
== system QuadcopterSimModel_INDI_Traj/Controller INDI/Multicopter INDI Loiter Flight Mode/Multicopter Altitude Hold Flight Mode with INDI and reduced attitude control ==
  cmd_roll_-1_1 : Inport  SampleTime=fm.sample_time
  cmd_pitch_-1_1 : Inport  Port=2  SampleTime=fm.sample_time
  cmd_yaw_rate_-1_1 : Inport  Port=3  SampleTime=fm.sample_time
  cmd_throttle_-1_1 : Inport  Port=4  SampleTime=fm.sample_time
  M_bg : Inport  Port=5  SampleTime=fm.sample_time
  omega_Kb : Inport  Port=6  SampleTime=fm.sample_time
  z_Kg : Inport  Port=7  SampleTime=fm.sample_time
  z_Kg_dt : Inport  Port=8  SampleTime=fm.sample_time
  initial_yaw : Inport  Port=9  SampleTime=fm.sample_time
  initial_z_Kg : Inport  Port=10  SampleTime=fm.sample_time
  is_cmd_in_NED : Inport  Port=11  SampleTime=fm.sample_time
  z-ref : Inport  Port=12
  manual_mode : Inport  Port=13
  yaw-ref : Inport  Port=14
  Add6 : Sum
  Bus Creator : BusCreator  Inputs=4
  Bus Selector : BusSelector  OutputSignals=pseudo_control.Delta_ny
  Bus Selector1 : BusSelector  OutputSignals=pseudo_control.Delta_ny
  Bus Selector6 : BusSelector  OutputSignals=x_ref
  Constant : Constant  Value=false(size(fm.ca.u_d))
  Delay : Delay  DelayLength=1
  Discrete Derivative : simulink/Discrete/Discrete Derivative  gainval=1.0  ICPrevScaledInput=0.0  OutMin=[]  OutMax=[]  OutDataType=fixdt(1, 16)  OutScaling=2^-10  DoSatur=off
  Discrete Derivative1 : simulink/Discrete/Discrete Derivative  gainval=1.0  ICPrevScaledInput=0.0  OutMin=[]  OutMax=[]  OutDataType=fixdt(1, 16)  OutScaling=2^-10  DoSatur=off
  INDI high level wls control allocation : control_allocation_lib/INDI high level wls control allocation for copters  ca=fm.ca
  MATLAB Function : MATLAB Function  TreatAsAtomicUnit=on
  MATLAB Function1 : MATLAB Function  TreatAsAtomicUnit=on
  Multicopter (Reduced) Attitude INDI Controller : Subsystem  AncestorBlock=cntrl_atti_red_indi_lib/Multicopter (Reduced) Attitude INDI Controller  mask{atti_cntrl=fm.cntrl.atti_cntrl, T=fm.motor_time_constant + 2./fm.sens_filt.omega}
      mask prompts: atti_cntrl "reduced attitude control struct"; T "inner loop time constant"
      mask Help: https://www.mathworks.com
      mask DialogControl DescGroupVar Prompt: INDI Reduced Attitude Controller
      mask DialogControl DescTextVar Prompt: To initialize the reduced attitude control struct see cntrlAttiRedIndiLoadParams
  Multicopter Altitude INDI Controller1 : Subsystem  AncestorBlock=cntrl_alt_indi/Multicopter Altitude INDI Controller  mask{alt_cntrl=fm.cntrl}
      mask prompts: alt_cntrl "reduced attitude control struct"
      mask DialogControl DescGroupVar Prompt: INDI Reduced Attitude Controller
      mask DialogControl DescTextVar Prompt: To initialize the reduced attitude control struct see cntrlAttiRedIndiLoadParams.
  Mux : Mux  Inputs=2
  PT1 discrete reference model : ndi_lib/PT1 discrete reference model  T=fm.motor_time_constant  x_max=inf  x_min=-inf  x_dt_max=inf  x_dt_min=-inf  x_init=0
      settings: SourceProductName=LADAC
  PT2 discrete with saturation1 : filters_lib/PT2 discrete with saturation  omega=fm.sens_filt.omega  d=fm.sens_filt.D  x_dt2_max=inf  x_dt2_min=-inf  x_dt_max=inf  x_dt_min=-inf  x_max=inf  x_min=-inf  x_init=0  x_dt_init=0
      settings: SourceProductName=LADAC
  Saturation3 : Saturate  UpperLimit=fm.ca.u_max  LowerLimit=fm.ca.u_min
  Terminator : Terminator
  Terminator1 : Terminator
  acceleration g to b frame : Subsystem
  control effectiveness : Subsystem
  fm_alt_hold : Outport  OutDataTypeStr=single  SampleTime=fm.sample_time
  wires:
  PT2 discrete with saturation1/1 -> Add6/2
  acceleration g to b frame/1(z_Kb_dt2_cmd) -> Mux/2
  M_bg/1 -> Multicopter (Reduced) Attitude INDI Controller/4(M_bg), acceleration g to b frame/2(M_bg)
  INDI high level wls control allocation/1 -> Add6/1, Bus Creator/4  "Delta_u"
  Mux/1 -> INDI high level wls control allocation/3
  cmd_pitch_-1_1/1 -> MATLAB Function1/2(stick_pitch_cmd)
  cmd_roll_-1_1/1 -> MATLAB Function1/1(stick_roll_cmd)
  Bus Creator/1 -> fm_alt_hold/1
  initial_z_Kg/1 -> Multicopter Altitude INDI Controller1/5(initial_z_Kg)
  Discrete Derivative1/1 -> Multicopter Altitude INDI Controller1/4(z_Kg_dt2)
  z_Kg_dt/1 -> Multicopter Altitude INDI Controller1/3(z_Kg_dt), Discrete Derivative1/1
  z_Kg/1 -> Multicopter Altitude INDI Controller1/2(z_Kg)
  PT2 discrete with saturation1/3 -> Terminator1/1
  PT2 discrete with saturation1/2 -> Terminator/1
  omega_Kb/1 -> Multicopter (Reduced) Attitude INDI Controller/5(omega_Kb), Discrete Derivative/1
  Discrete Derivative/1 -> Multicopter (Reduced) Attitude INDI Controller/6(omega_Kb_dt)
  Bus Selector/1 -> Mux/1  "<Delta_ny>"
  MATLAB Function1/1(lean_angle) -> Multicopter (Reduced) Attitude INDI Controller/1(cmd_lean_angle_0_1)
  initial_yaw/1 -> Multicopter (Reduced) Attitude INDI Controller/7(initial_yaw)
  Multicopter (Reduced) Attitude INDI Controller/1(atti_cntrl) -> Bus Selector/1, Bus Creator/2  "atti_cntrl"
  Bus Selector6/1 -> Delay/1, control effectiveness/1(u), INDI high level wls control allocation/4  "<x_ref>"
  control effectiveness/2(G2) -> INDI high level wls control allocation/2
  Add6/1 -> Saturation3/1
  cmd_throttle_-1_1/1 -> Multicopter Altitude INDI Controller1/1(cmd_throttle_-1_1), MATLAB Function/1(u)
  MATLAB Function/1(y) -> INDI high level wls control allocation/5  "throttle_0_1"
  Bus Selector1/1 -> acceleration g to b frame/1(z_Kg_dt2_cmd)  "<Delta_ny>"
  MATLAB Function1/2(lean_direction_angle) -> Multicopter (Reduced) Attitude INDI Controller/2(cmd_lean_direction_angle_0_2pi)
  Delay/1 -> PT2 discrete with saturation1/1
  Constant/1 -> INDI high level wls control allocation/6
  PT1 discrete reference model/1 -> Bus Selector6/1
  Saturation3/1 -> PT1 discrete reference model/1, Bus Creator/3  "u"
  cmd_yaw_rate_-1_1/1 -> Multicopter (Reduced) Attitude INDI Controller/3(cmd_yaw_rate_-1_1)
  Multicopter Altitude INDI Controller1/1(alt_cntrl) -> Bus Selector1/1, Bus Creator/1  "alt_cntrl"
  control effectiveness/1(G1) -> INDI high level wls control allocation/1
  is_cmd_in_NED/1 -> Multicopter (Reduced) Attitude INDI Controller/8(is_cmd_in_NED)
  z-ref/1 -> Multicopter Altitude INDI Controller1/6(z_Ref)
  manual_mode/1 -> Multicopter (Reduced) Attitude INDI Controller/10(manual_mode), Multicopter Altitude INDI Controller1/7(manual_mode)
  yaw-ref/1 -> Multicopter (Reduced) Attitude INDI Controller/9("yaw_ref ")

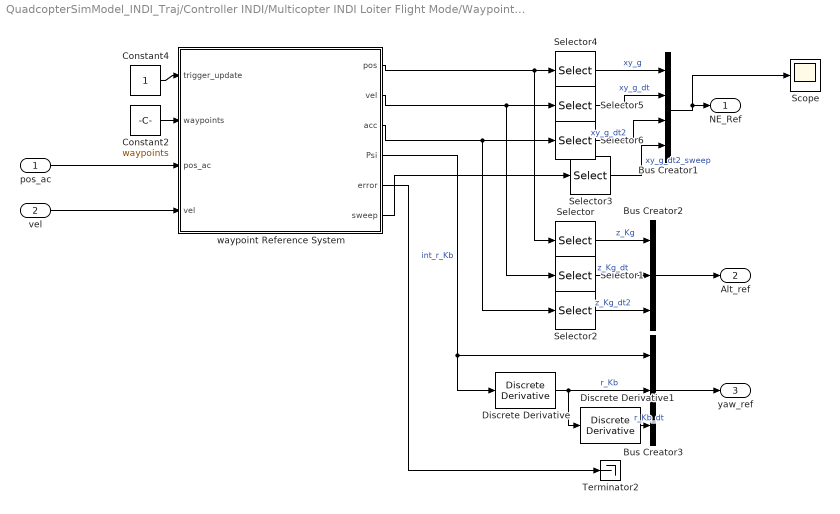
== system QuadcopterSimModel_INDI_Traj/Controller INDI/Multicopter INDI Loiter Flight Mode/Waypoint Reference ==
  pos_ac : Inport
  vel : Inport  Port=2
  Bus Creator1 : BusCreator  Inputs=4
  Bus Creator2 : BusCreator  Inputs=3
  Bus Creator3 : BusCreator  Inputs=3
  Constant2 : Constant  Value=waypoints
  Constant4 : Constant  OutDataTypeStr=boolean
  Discrete Derivative : simulink/Discrete/Discrete Derivative  gainval=1  ICPrevScaledInput=0.0  OutMin=[]  OutMax=[]  OutDataType=fixdt(1, 16)  OutScaling=2^-10  DoSatur=off
  Discrete Derivative1 : simulink/Discrete/Discrete Derivative  gainval=1  ICPrevScaledInput=0.0  OutMin=[]  OutMax=[]  OutDataType=fixdt(1, 16)  OutScaling=2^-10  DoSatur=off
  Scope : Scope
  Selector : Selector  InputPortWidth=3  IndexOptions=Index vector (dialog)  Indices=3  OutputSizes=1
  Selector1 : Selector  InputPortWidth=3  IndexOptions=Index vector (dialog)  Indices=3  OutputSizes=1
  Selector2 : Selector  InputPortWidth=3  IndexOptions=Index vector (dialog)  Indices=3  OutputSizes=1
  Selector{3..6} (4 alike) : Selector  InputPortWidth=3  IndexOptions=Index vector (dialog)  Indices=[1 2]  OutputSizes=1
  Terminator2 : Terminator
  waypoint Reference System : Subsystem
  NE_Ref : Outport
  Alt_ref : Outport  Port=2
  yaw_ref : Outport  Port=3
  wires:
  waypoint Reference System/2(vel) -> Selector1/1, Selector5/1
  Selector6/1 -> Bus Creator1/3  "xy_g_dt2"
  Bus Creator1/1 -> Scope/1, NE_Ref/1
  waypoint Reference System/1(pos) -> Selector/1, Selector4/1
  Selector4/1 -> Bus Creator1/1  "xy_g"
  waypoint Reference System/3(acc) -> Selector2/1, Selector6/1
  Constant4/1 -> waypoint Reference System/1(trigger_update)
  Selector5/1 -> Bus Creator1/2  "xy_g_dt"
  Constant2/1 -> waypoint Reference System/2(waypoints)
  waypoint Reference System/5(error) -> Terminator2/1
  waypoint Reference System/4(Psi) -> Discrete Derivative/1, Bus Creator3/1  "int_r_Kb"
  Selector/1 -> Bus Creator2/1  "z_Kg"
  Selector1/1 -> Bus Creator2/2  "z_Kg_dt"
  Selector2/1 -> Bus Creator2/3  "z_Kg_dt2"
  Bus Creator2/1 -> Alt_ref/1
  pos_ac/1 -> waypoint Reference System/3(pos_ac)
  Bus Creator3/1 -> yaw_ref/1
  Discrete Derivative/1 -> Discrete Derivative1/1, Bus Creator3/2  "r_Kb"
  Discrete Derivative1/1 -> Bus Creator3/3  "r_Kb_dt"
  vel/1 -> waypoint Reference System/4("vel ")
  waypoint Reference System/6("sweep ") -> Selector3/1
  Selector3/1 -> Bus Creator1/4  "xy_g_dt2_sweep"

== system QuadcopterSimModel_INDI_Traj/Controller INDI/Multicopter INDI Loiter Flight Mode/command direction ==
  cmd_u_-1_1 : Inport
  cmd_v_-1_1 : Inport  Port=2
  is_cmd_in_NED : Inport  Port=3
  M_bg : Inport  Port=4
  MATLAB Function : MATLAB Function  TreatAsAtomicUnit=on
  cmd_north_vel_-1_1 : Outport
  cmd_east_vel_-1_1 : Outport  Port=2
  wires:
  M_bg/1 -> MATLAB Function/4(M_bg)
  MATLAB Function/2(cmd_v_E) -> cmd_east_vel_-1_1/1
  MATLAB Function/1(cmd_u_N) -> cmd_north_vel_-1_1/1
  is_cmd_in_NED/1 -> MATLAB Function/3(is_NED)
  cmd_v_-1_1/1 -> MATLAB Function/2(cmd_v)
  cmd_u_-1_1/1 -> MATLAB Function/1(cmd_u)

== system QuadcopterSimModel_INDI_Traj/Controller INDI/filtering/PT2 discrete with saturation3 ==
  u : Inport
  u0 : Inport  Port=2
  2*d/omega : Gain  Gain=2*d./omega
  Discrete-Time Integrator y : DiscreteIntegrator  InitialConditionSource=external  InitialCondition=x_init  SampleTime=-1  OutDataTypeStr=Inherit: Inherit via back propagation  LimitOutput=on  UpperSaturationLimit=x_max  LowerSaturationLimit=x_min  ICPrevOutput=DiscIntNeverNeededParam  ICPrevScaledInput=DiscIntNeverNeededParam
  Discrete-Time Integrator y_dt : DiscreteIntegrator  InitialCondition=x_dt_init  SampleTime=-1  OutDataTypeStr=Inherit: Inherit via back propagation  LimitOutput=on  UpperSaturationLimit=x_dt_max  LowerSaturationLimit=x_dt_min  ICPrevOutput=DiscIntNeverNeededParam  ICPrevScaledInput=DiscIntNeverNeededParam
  Saturation : Saturate  UpperLimit=x_dt2_max  LowerLimit=x_dt2_min
  Sum2 : Sum  Inputs=|+-
  Sum3 : Sum  Inputs=|++
  omega^2 : Gain  Gain=omega.^2
  y : Outport
  y_dt : Outport  Port=2
  y_dt2 : Outport  Port=3
  wires:
  Saturation/1 -> y_dt2/1, Discrete-Time Integrator y_dt/1  "y_dt2"
  omega^2/1 -> Saturation/1
  Sum3/1 -> Sum2/2
  u/1 -> Sum2/1
  2*d/omega/1 -> Sum3/2
  Sum2/1 -> omega^2/1
  Discrete-Time Integrator y/1 -> Sum3/1, y/1  "y"
  Discrete-Time Integrator y_dt/1 -> 2*d/omega/1, y_dt/1, Discrete-Time Integrator y/1  "y_dt"
  u0/1 -> Discrete-Time Integrator y/2

== system QuadcopterSimModel_INDI_Traj/stick inputs/Signal builder/Signal Builder ==
  Demux : Demux  Tag=STV Demux  Outputs=1
  FromWs : FromWorkspace  Tag=STV FromWs  VariableName=tuvar  SampleTime=0
      SigBuilderData=|
      | common.afterFinalStr = 'Extrapolate'
      | common.sampleTime = 0
      | dataSet.timeRange = [0 10]
      | dataSet.name = 'Group 1'
      | sbobj.Groups.Name = 'Group 1'
      | sbobj.Groups.Signals.Name = 'Signal 1'
      | sbobj.Groups.Signals.XData = [0 8 8 9.9 9.9 9.92 9.92 9.96 9.96 10]
      | sbobj.Groups.Signals.YData = [0 0 1 1 1.005 0.803 0.8 0.4 0 0]
  Signal 1 : Outport  Tag=STV Outport
  wires:
  Demux/1 -> Signal 1/1
  FromWs/1 -> Demux/1

== system QuadcopterSimModel_INDI_Traj/stick inputs/Signal builder/Signal Builder1 ==
  Demux : Demux  Tag=STV Demux  Outputs=1
  FromWs : FromWorkspace  Tag=STV FromWs  VariableName=tuvar  SampleTime=0
      SigBuilderData=|
      | common.afterFinalStr = 'Extrapolate'
      | common.sampleTime = 0
      | dataSet.timeRange = [0 10]
      | dataSet.name = 'Group 1'
      | sbobj.Groups.Name = 'Group 1'
      | sbobj.Groups.Signals.Name = 'Signal 1'
      | sbobj.Groups.Signals.XData = [0 4 4 6 6 10]
      | sbobj.Groups.Signals.YData = [0 0 1 1 0 0]
  Signal 1 : Outport  Tag=STV Outport
  wires:
  Demux/1 -> Signal 1/1
  FromWs/1 -> Demux/1
